simulink model "Fig310"  (Simulink 8.4)
settings: Solver=ode3  StartTime=0.0  StopTime=5.24288  FixedStep=2e-6  RelTol=1e-5
libraries: commanapbnd3 x1, commrandsrc2 x1
settings Model: Creator=Dennis Silage  LastModifiedBy=Silage
settings OptimizationCC: InitFltsAndDblsToZero=on
settings DebuggingCC: SolverPrmCheckMsg=none

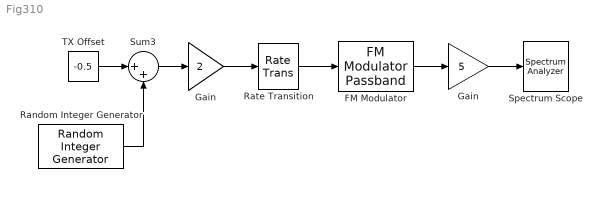
== system Fig310 ==
  FM Modulator : commanapbnd3/FM Modulator Passband  Fc=20000  Ph=0  Kc=500
  Gain : Gain  Gain=2
  "Gain " : Gain  Gain=5
  Random Integer Generator : commrandsrc2/Random Integer Generator  mul=2  seed=randseed  Ts=1e-3  frameBased=off  sampPerFrame=50  orient=on  outDataType=double
  Rate Transition : RateTransition  OutPortSampleTime=2e-6
  Spectrum Scope : SpectrumAnalyzer
  Sum3 : Sum  Inputs=|++
  TX Offset : Constant  Value=-0.5
  wires:
  Sum3/1 -> Gain/1
  TX Offset/1 -> Sum3/1
  Random Integer Generator/1 -> Sum3/2
  Rate Transition/1 -> FM Modulator/1
  Gain/1 -> Rate Transition/1
  FM Modulator/1 -> "Gain "/1
  "Gain "/1 -> Spectrum Scope/1
